simulink model "modelo_planta_CODESYS_EXPERIMENTAL"  (R2025b)
settings: Solver=FixedStepAuto  StartTime=0.0  StopTime=inf  FixedStep=Ts2  MaxStep=1e-3  RelTol=1e-3
undefined symbols (not defined in the file): ah_max, at_max, bcx, bcy, bh_eq, bhb, bhEb, bhwu, bt, bt_eq, btb, btw, g, Hc, ih, it, Jh_eq, Jt_eq, Kcy, khwu, Ki_h, Ki_t, Kp_h, Kp_t, Ktw, lambda, Lh, Lh0, lh_0, Lt, magnitude, Mc_max, Ms, Mt, rhd, rtd, tau_hm, tau_tm, Thb_Max, ThEb_Max, Thm_0, Thm_Max, titahm_0, titatm_0, Ts0, Ts1, Ts2, Ttb_Max, Ttm_0, Ttm_Max, vh_0, vlx_0, vly_0, vt_0, vt_max, Wc, whm_0, whm_rated, wtm_0, xl_0 ... (+9)
libraries: simulink x10, opcualib x9, sl3dlib x1, simulink_extras x1, dspnetwork x1
(part 2 of 2)

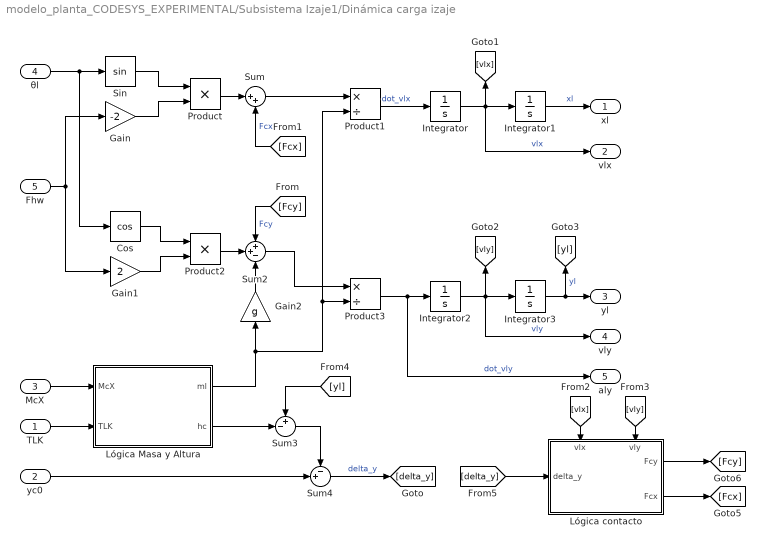
== system modelo_planta_CODESYS_EXPERIMENTAL/Subsistema Izaje1/Dinámica carga izaje ==
  TLK : Inport
  yc0 : Inport  Port=2
  McX : Inport  Port=3
  θl : Inport  Port=4
  Fhw : Inport  Port=5
  Cos : Trigonometry  Operator=cos
  Gain : Gain  Gain=-2
  Gain1 : Gain  Gain=2
  Gain2 : Gain  Gain=g
  Integrator : Integrator  InitialCondition=vlx_0
  Integrator1 : Integrator  InitialCondition=xl_0
  Integrator2 : Integrator  InitialCondition=vly_0
  Integrator3 : Integrator  InitialCondition=yl_0
  Lógica Masa y Altura : Subsystem
  Lógica contacto : Subsystem
      settings: PortSchema="{\"entries\":[{\"content\":{\"sides\":[{\"content\":{\"connectorIds\":[\"In1\"]},\"type\":\"ConnectorPlacement.EquallySpacedRectSide\",\"uuid\":\"20a8b2c4-d5cf-44ce-93ec-929b996a0905\"},{\"content\":{\"connectorIds\":[\"Out1\",\"Out2\"],\"side\":\"RIGHT\"},\"type\":\"ConnectorPlacement.EquallySpacedRectSide\",\"uuid\":\"396e1f2e-cf71-48dc-8d57-a3e2695dfff1\"},{\"content\":{\"connectorIds\":[\"In2\",\"In3\"],\"side\":\"TOP\"},\"type\":\"ConnectorPlacement.EquallySpacedRectSide\",\"uuid\":\"e66c0478-9682-41e1-9b77-d2d789a9c323\"}]},\"type\":\"ConnectorPlacement.EquallySpacedConnector\",\"uuid\":\"193dabd2-f524-433a-b6ef-c1cab585578e\"}],\"packageUris\":[\"http://schema.mathworks.com/mf0/Connector/R2020b\"],\"version\":\"1.0\"}"
  Product : Product
  Product1 : Product  Inputs=*/
  Product2 : Product
  Product3 : Product  Inputs=*/
  Sin : Trigonometry
  Sum : Sum  Inputs=|++
  Sum2 : Sum  Inputs=++-
  Sum3 : Sum  Inputs=+-|
  Sum4 : Sum  Inputs=-+|
  xl : Outport
  vlx : Outport  Port=2
  yl : Outport  Port=3
  vly : Outport  Port=4
  aly : Outport  Port=5
  wires:
  θl/1 -> Sin/1, Cos/1
  Integrator/1 -> vlx/1, Integrator1/1, [vlx]  "vlx"
  Sum3/1 -> Sum4/1
  Sin/1 -> Product/1
  Gain/1 -> Product/2
  [Fcy] -> Sum2/1  "Fcy"
  Integrator2/1 -> vly/1, Integrator3/1, [vly]  "vly"
  Integrator3/1 -> yl/1, [yl]  "yl"
  Fhw/1 -> Gain1/1, Gain/1
  [Fcx] -> Sum/2  "Fcx"
  Product/1 -> Sum/1
  Product1/1 -> Integrator/1  "dot_vlx"
  Gain2/1 -> Sum2/3
  Cos/1 -> Product2/1
  Gain1/1 -> Product2/2
  [yl] -> Sum3/1
  Product2/1 -> Sum2/2
  yc0/1 -> Sum4/2
  Sum2/1 -> Product3/1
  Product3/1 -> aly/1, Integrator2/1  "dot_vly"
  Sum/1 -> Product1/1
  Integrator1/1 -> xl/1  "xl"
  Sum4/1 -> [delta_y]  "delta_y"
  Lógica contacto/1(Fcy) -> [Fcy]
  Lógica contacto/2(Fcx) -> [Fcx]
  Lógica Masa y Altura/1(ml) -> Product1/2, Product3/2, Gain2/1
  McX/1 -> Lógica Masa y Altura/1(McX)
  TLK/1 -> Lógica Masa y Altura/2(TLK)
  Lógica Masa y Altura/2(hc) -> Sum3/2
  [vlx] -> Lógica contacto/2(vlx)
  [vly] -> Lógica contacto/3(vly)
  [delta_y] -> Lógica contacto/1(delta_y)

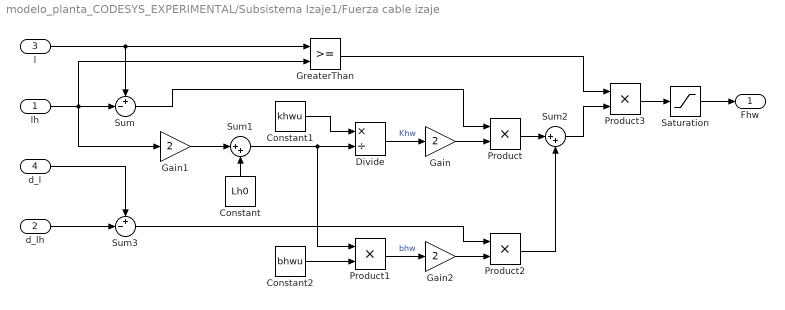
== system modelo_planta_CODESYS_EXPERIMENTAL/Subsistema Izaje1/Fuerza cable izaje ==
  lh : Inport
  d_lh : Inport  Port=2
  l : Inport  Port=3
  d_l : Inport  Port=4
  Constant : Constant  Value=Lh0
  Constant1 : Constant  Value=khwu
  Constant2 : Constant  Value=bhwu
  Divide : Product  Inputs=*/  RndMeth=Zero  SaturateOnIntegerOverflow=on
  Gain : Gain  Gain=2
  Gain1 : Gain  Gain=2
  Gain2 : Gain  Gain=2
  GreaterThan : RelationalOperator  OutDataTypeStr=boolean  RndMeth=Simplest  InputSameDT=off
  Product{,1..3} (4 alike) : Product
  Saturation : Saturate  UpperLimit=inf  LowerLimit=0
  Sum : Sum  Inputs=+-|
  Sum1 : Sum  Inputs=|++
  Sum2 : Sum  Inputs=|++
  Sum3 : Sum  Inputs=+-|
  Fhw : Outport
  wires:
  Constant/1 -> Sum1/2
  Constant2/1 -> Product1/2
  Sum1/1 -> Divide/2, Product1/1
  lh/1 -> Sum/2, GreaterThan/2, Gain1/1
  Product/1 -> Sum2/1
  Gain1/1 -> Sum1/1
  l/1 -> Sum/1, GreaterThan/1
  Product2/1 -> Sum2/2
  Product3/1 -> Saturation/1
  GreaterThan/1 -> Product3/1
  d_lh/1 -> Sum3/2
  Constant1/1 -> Divide/1
  Product1/1 -> Gain2/1  "bhw"
  Sum/1 -> Product/1
  Gain2/1 -> Product2/2
  Divide/1 -> Gain/1  "Khw"
  Sum2/1 -> Product3/2
  Sum3/1 -> Product2/1
  d_l/1 -> Sum3/1
  Gain/1 -> Product/2
  Saturation/1 -> Fhw/1

== system modelo_planta_CODESYS_EXPERIMENTAL/Subsistema Carro1/Accionamiento carro/Freno Motor ==
  BRK_t : Inport
  wtm : Inport  Port=2
  Constant : Constant  Value=0
  Gain3 : Gain  Gain=-Ttb_Max
  Gain4 : Gain  Gain=btb
  Switch : Switch  Criteria=u2 > Threshold  SaturateOnIntegerOverflow=off  InputSameDT=off
  Tanh : Trigonometry  Operator=tanh
  Ttb : Outport
  wires:
  BRK_t/1 -> Switch/2
  Constant/1 -> Switch/1
  wtm/1 -> Gain4/1
  Gain4/1 -> Tanh/1
  Tanh/1 -> Gain3/1
  Gain3/1 -> Switch/3
  Switch/1 -> Ttb/1

== system modelo_planta_CODESYS_EXPERIMENTAL/Subsistema Izaje1/Accionamiento izaje/Freno Emergencia (Drum) ==
  BRK_hE : Inport
  whd : Inport  Port=2
  Constant : Constant  Value=0
  Gain3 : Gain  Gain=-ThEb_Max
  Gain4 : Gain  Gain=bhEb
  Switch : Switch  Criteria=u2 > Threshold  SaturateOnIntegerOverflow=off  InputSameDT=off
  Tanh : Trigonometry  Operator=tanh
  ThEb : Outport
  wires:
  BRK_hE/1 -> Switch/2
  Gain3/1 -> Switch/3
  Constant/1 -> Switch/1
  whd/1 -> Gain4/1
  Gain4/1 -> Tanh/1
  Tanh/1 -> Gain3/1
  Switch/1 -> ThEb/1

== system modelo_planta_CODESYS_EXPERIMENTAL/Subsistema Izaje1/Accionamiento izaje/Freno Motor ==
  BRK_h : Inport
  whm : Inport  Port=2
  Constant : Constant  Value=0
  Gain3 : Gain  Gain=-Thb_Max
  Gain4 : Gain  Gain=bhb
  Switch : Switch  Criteria=u2 > Threshold  SaturateOnIntegerOverflow=off  InputSameDT=off
  Tanh : Trigonometry  Operator=tanh
  Thb : Outport
  wires:
  BRK_h/1 -> Switch/2
  Gain3/1 -> Switch/3
  Constant/1 -> Switch/1
  whm/1 -> Gain4/1
  Gain4/1 -> Tanh/1
  Tanh/1 -> Gain3/1
  Switch/1 -> Thb/1

== system modelo_planta_CODESYS_EXPERIMENTAL/Subsistema Izaje1/Dinámica carga izaje/Lógica Masa y Altura ==
  McX : Inport
  TLK : Inport  Port=2
  Constant : Constant  Value=Ms
  Constant1 : Constant  Value=0
  Constant2 : Constant  Value=Hc
  Rate Limiter : RateLimiter  Commented=through  RisingSlewLimit=Mc_max/0.1  FallingSlewLimit=-Mc_max/0.1  SampleTimeMode=inherited  InitialCondition=Ms
  Sum1 : Sum  Inputs=|++
  Switch : Switch  Criteria=u2 > Threshold  SaturateOnIntegerOverflow=off  InputSameDT=off
  Switch1 : Switch  Criteria=u2 > Threshold  SaturateOnIntegerOverflow=off  InputSameDT=off
  ml : Outport
  hc : Outport  Port=2
  wires:
  Sum1/1 -> Switch/1
  Constant2/1 -> Switch1/1
  TLK/1 -> Switch1/2, Switch/2
  Constant/1 -> Switch/3, Sum1/2
  Constant1/1 -> Switch1/3
  McX/1 -> Sum1/1
  Switch/1 -> Rate Limiter/1
  Rate Limiter/1 -> ml/1
  Switch1/1 -> hc/1

== system modelo_planta_CODESYS_EXPERIMENTAL/Subsistema Izaje1/Dinámica carga izaje/Lógica contacto ==
  delta_y : Inport
  vlx : Inport  Port=2
  vly : Inport  Port=3
  Constant3 : Constant  Value=0
  Constant4 : Constant  Value=0
  Gain3 : Gain  Gain=Kcy
  Gain4 : Gain  Gain=bcy
  Gain5 : Gain  Gain=-bcx
  Saturation : Saturate  UpperLimit=60e5  LowerLimit=0
  Sum5 : Sum  Inputs=-+|
  Switch2 : Switch  SaturateOnIntegerOverflow=off  InputSameDT=off
  Switch3 : Switch  SaturateOnIntegerOverflow=off  InputSameDT=off
  Fcy : Outport
  Fcx : Outport  Port=2
  wires:
  Sum5/1 -> Switch2/1
  vlx/1 -> Gain5/1
  Gain4/1 -> Sum5/1
  vly/1 -> Gain4/1
  Constant4/1 -> Switch3/3
  Gain5/1 -> Switch3/1
  Gain3/1 -> Sum5/2
  delta_y/1 -> Switch3/2, Gain3/1, Switch2/2
  Constant3/1 -> Switch2/3
  Switch2/1 -> Saturation/1  "Fcy"
  Switch3/1 -> Fcx/1  "Fcx"
  Saturation/1 -> Fcy/1

== matlab function modelo_planta_CODESYS_EXPERIMENTAL/Controlador Izaje2/MATLAB Function1 ==
  data: m_est input; Thm_ref output; vh_ref input; vh_obs input; BRK input; ih parameter; rhd parameter; g parameter; Kp_h parameter; Ki_h parameter; Ts2 parameter
function Thm_ref = ControladorDeVelocidad(m_est, vh_ref, vh_obs, BRK, ih, rhd, g, Kp_h, Ki_h, Ts2)
persistent int_prev e_w_prev

if isempty(int_prev)
    int_prev = 0.0;
    e_w_prev = 0.0;
end

e_w = (vh_ref - vh_obs) * (2 * ih / rhd);

if BRK > 0
    int_val = int_prev + (Ts2 / 2) * (e_w + e_w_prev);
else
    int_val = 0.0;
    e_w_prev = 0.0;
end

T_PID = Kp_h * e_w + Ki_h * int_val;
Tg_ff = m_est * (g * rhd / (2 * ih));

Thm_ref = T_PID + Tg_ff;

int_prev = int_val;
e_w_prev = e_w;
end

== matlab function modelo_planta_CODESYS_EXPERIMENTAL/Controlador Izaje2/MATLAB Function3 ==
  data: yh_enc input; vh_obs output; Thm_ref input; whm_0 parameter; titahm_0 parameter; Lh parameter; bh_eq parameter; Jh_eq parameter; rhd parameter; ih parameter; Ts2 parameter; Ms parameter; g parameter
function vh_obs = Observador_Estado_h(yh_enc, Thm_ref, whm_0, titahm_0,...
    Lh, bh_eq, Jh_eq, rhd, ih, Ts2, Ms, g)
    
    % Memorias
    persistent theta_h_obs_prev wh_obs_prev int_e_prev
    
    % Condiciones iniciales
    if isempty(theta_h_obs_prev)
        theta_h_obs_prev = titahm_0;
        wh_obs_prev      = whm_0;    
        int_e_prev       = 0.0; 
    end
    
    % 1. Convertir posición lineal del carro a angular del motor
    theta_h_enc = yh_enc * (2*ih / rhd);
    
    % 2. Error de estimación (Posición real vs observada)
    e_theta_h = theta_h_enc - theta_h_obs_prev;
    
    % 3. Lazo de torque (Física de la planta)
    Torque_net = Thm_ref - (Ms*g*rhd/(2*ih)) - (bh_eq * wh_obs_prev) +...
        (Lh(3) * int_e_prev);
    alpha_phys = Torque_net / Jh_eq; % Aceleración angular
    
    % 4. Derivadas
    dot_wh_obs      = alpha_phys + (Lh(2) * e_theta_h);
    dot_theta_h_obs = wh_obs_prev + (Lh(1) * e_theta_h);

    % 5. Salida del observador
    vh_obs = wh_obs_prev * (rhd / (2*ih));
    
    % 6. Integración Discreta
    theta_h_obs = theta_h_obs_prev + (Ts2 * dot_theta_h_obs);
    wh_obs      = wh_obs_prev      + (Ts2 * dot_wh_obs);
    int_e       = int_e_prev       + (Ts2 * e_theta_h);

    % 7. Actualizar memorias para el siguiente ciclo de reloj
    theta_h_obs_prev = theta_h_obs;
    wh_obs_prev      = wh_obs;
    int_e_prev       = int_e;
end

== matlab function modelo_planta_CODESYS_EXPERIMENTAL/MATLAB Function ==
  data: TLK input; M_carga output; Mc_min parameter
function M_carga = Masa_Aleatoria(TLK, Mc_min)
    persistent masa_actual;
    persistent ultimo_estado_trigger;
    
    % Inicialización
    if isempty(masa_actual)
        masa_actual = Mc_min; % Empezamos con el valor mínimo por defecto
        ultimo_estado_trigger = 0;
    end
    
    % DETECCIÓN DE FLANCO DE SUBIDA (Rising Edge)
    if (TLK == 1 && ultimo_estado_trigger == 0)
        % Generar número aleatorio entre Min y Max
        masa_actual = Mc_min + (55000 - Mc_min) * rand();
        masa_actual = floor(masa_actual); 
    end
    
    % Actualizar memoria del trigger
    ultimo_estado_trigger = TLK;
    % Salida: La masa se mantiene constante hasta el próximo trigger
    M_carga = masa_actual;
end

== matlab function modelo_planta_CODESYS_EXPERIMENTAL/MATLAB Function1 ==
  data: yc0 output; xl input; xt_min parameter; Wc parameter; h_vec input
function yc0 = Y_spreader(xl, xt_min, Wc, h_vec)
% Cálculo índice de spreader
i_spreader = floor((xl - xt_min)/Wc) + 1;
i_spreader = min(max(i_spreader, 1), 33);

% Obtención de yc0 usando la posición del spreader
yc0 = h_vec(i_spreader);

== matlab function modelo_planta_CODESYS_EXPERIMENTAL/Controlador Carro2/MATLAB Function ==
  data: tita_l input; v_sway output; yh_enc input; anti_sway input; Yt0 parameter; g parameter; lambda parameter
function v_sway = ControlDeBalanceo(tita_l, yh_enc, anti_sway, Yt0, g, lambda)

lh = abs(Yt0-yh_enc);

K_sway = 2 *lambda * sqrt(g*lh);

if(anti_sway)
    v_sway = K_sway * tita_l;
else
    v_sway = 0;
end

== matlab function modelo_planta_CODESYS_EXPERIMENTAL/Controlador Carro2/MATLAB Function1 ==
  data: vx_cmd input; seleccion input; vt_ref output; v_sway input; Ts2 parameter; at_max parameter; vt_max parameter; vt_0 parameter
function vt_ref = ModulacionDeLaReferencia(vx_cmd, seleccion, v_sway, Ts2, at_max, vt_max, vt_0)

persistent vt_ref_prev

if isempty(vt_ref_prev)
    vt_ref_prev = vt_0;
end

if seleccion > 0
    vel_base = 0;
else
    vel_base = vx_cmd;
end

vt_cmd = vel_base + v_sway;
vt_cmd_sat = min(max(vt_cmd, -vt_max), vt_max);

delta_v = vt_cmd_sat - vt_ref_prev;
limite_delta = at_max * Ts2;
delta_v_limitado = min(max(delta_v, -limite_delta), limite_delta);

vt_ref = vt_ref_prev + delta_v_limitado;
vt_ref_prev = vt_ref;

== matlab function modelo_planta_CODESYS_EXPERIMENTAL/Controlador Carro2/MATLAB Function3 ==
  data: xtd_enc input; vt_obs output; Ttm_ref input; wtm_0 parameter; titatm_0 parameter; Lt parameter; bt_eq parameter; Jt_eq parameter; rtd parameter; it parameter; Ts2 parameter
function vt_obs = Observador_Estado_t(xtd_enc, Ttm_ref, wtm_0, titatm_0, Lt, bt_eq, Jt_eq, rtd, it, Ts2)...
    
    % Memorias
    persistent theta_t_obs_prev wt_obs_prev int_e_prev
    
    % Condiciones iniciales
    if isempty(theta_t_obs_prev)
        theta_t_obs_prev = titatm_0;
        wt_obs_prev      = wtm_0;    
        int_e_prev       = 0.0; 
    end
    
    % 1. Convertir posición lineal del carro a angular del motor
    theta_t_enc = xtd_enc * (it / rtd);
    
    % 2. Error de estimación (Posición real vs observada)
    e_theta_t = theta_t_enc - theta_t_obs_prev;
    
    % 3. Lazo de torque (Física de la planta)
    Torque_net = Ttm_ref - (bt_eq * wt_obs_prev) + (Lt(3) * int_e_prev);
    alpha_phys = Torque_net / Jt_eq; % Aceleración angular
    
    % 4. Derivadas
    dot_wt_obs      = alpha_phys + (Lt(2) * e_theta_t);
    dot_theta_t_obs = wt_obs_prev + (Lt(1) * e_theta_t);

    % 5. Salida del observador
    vt_obs = wt_obs_prev * (rtd / it);
    
    % 6. Integración Discreta
    theta_t_obs = theta_t_obs_prev + (Ts2 * dot_theta_t_obs);
    wt_obs      = wt_obs_prev      + (Ts2 * dot_wt_obs);
    int_e       = int_e_prev       + (Ts2 * e_theta_t);

    % 7. Actualizar memorias para el siguiente ciclo de reloj
    theta_t_obs_prev = theta_t_obs;
    wt_obs_prev      = wt_obs;
    int_e_prev       = int_e;
end

== matlab function modelo_planta_CODESYS_EXPERIMENTAL/Controlador Carro2/MATLAB Function4 ==
  data: vt_ref input; Ttm_ref output; vt_obs input; BRK_t input; Ts2 parameter; Ki_t parameter; Kp_t parameter
function Ttm_ref = ControladorDeVelocidad(vt_ref, vt_obs, BRK_t, Ts2, Ki_t, Kp_t)
    % Memorias para el integrador
    persistent int_prev e_v_prev
    
    % Inicialización
    if isempty(int_prev)
        int_prev = 0.0;
        e_v_prev = 0.0;
    end
    
    % 1. Cálculo del error de velocidad
    e_v = vt_ref - vt_obs;
    
    % 2. Integrador Discreto (Tustin) con Reset por Freno
    % Si el freno está activo (BRK_t = 0), forzamos la memoria a 0 
    % para evitar la acumulación de error (Anti-Windup).
    if BRK_t > 0
        int_val = int_prev + (Ts2 / 2) * (e_v + e_v_prev);
    else
        int_val = 0.0;
    end
    
    % 3. Controlador PI
    P_out = e_v * Kp_t;
    I_out = int_val * Ki_t;
    
    % Suma final de referencia de torque
    Ttm_ref = P_out + I_out;
    
    % 4. Actualizar memorias
    int_prev = int_val;
    e_v_prev = e_v;
end

== matlab function modelo_planta_CODESYS_EXPERIMENTAL/Controlador Izaje2/MATLAB Function ==
  data: vy_cmd input; vh_ref output; seleccion input; ah_max parameter; Ts2 parameter; vh_0 parameter; vh_lim input
function vh_ref = ModulacionDeLaReferencia(vy_cmd, seleccion, ah_max, Ts2, vh_0, vh_lim)
persistent vh_ref_prev

if isempty(vh_ref_prev)
    vh_ref_prev = vh_0;
end

if seleccion > 0
    vh_cmd = 0;
else
    vh_cmd = vy_cmd;
end

vh_cmd_sat = min(max(vh_cmd, -vh_lim), vh_lim);

delta_v = vh_cmd_sat - vh_ref_prev;
limite_delta = ah_max * Ts2;
delta_v_limitado = min(max(delta_v, -limite_delta), limite_delta);

vh_ref = vh_ref_prev + delta_v_limitado;
vh_ref_prev = vh_ref;
end
